simulink model "LoadTransferModel"  (R2026b)
settings: Solver=ode45  StopTime=1
undefined symbols (not defined in the file): Simulation, Vehicle
settings Model: DataDictionary=VehicleData.sldd  Creator=Xu Dingyi  LastModifiedBy=29358

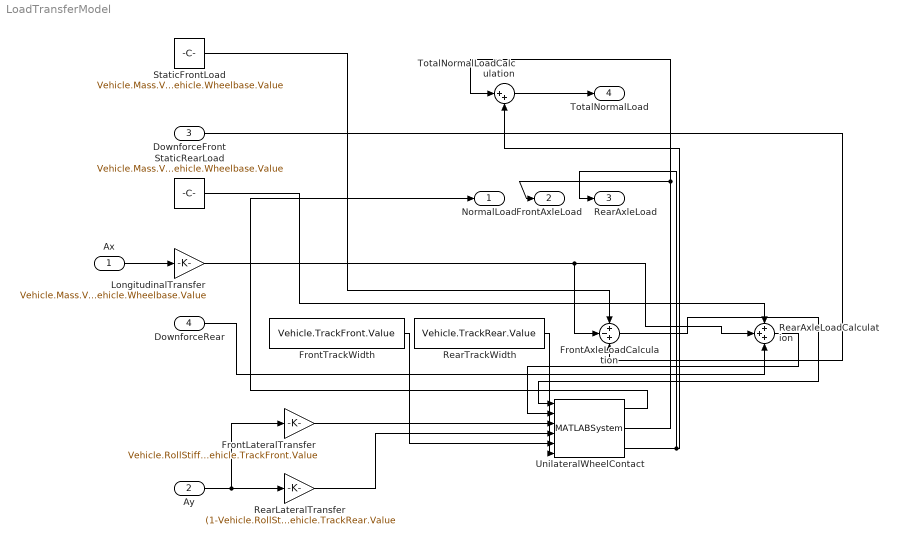
== system LoadTransferModel ==
  Ax : Inport  OutDataTypeStr=double  PortDimensions=1
  Ay : Inport  Port=2  OutDataTypeStr=double  PortDimensions=1
  DownforceFront : Inport  Port=3  OutDataTypeStr=double  PortDimensions=1
  DownforceRear : Inport  Port=4  OutDataTypeStr=double  PortDimensions=1
  FrontAxleLoadCalculation : Sum  Inputs=+-+
  FrontLateralTransfer : Gain  Gain=Vehicle.RollStiffnessDistributionFront.Value*Vehicle.Mass.Value*Vehicle.CGHeight.Value/Vehicle.TrackFront.Value
  FrontTrackWidth : Constant  Value=Vehicle.TrackFront.Value
  LongitudinalTransfer : Gain  Gain=Vehicle.Mass.Value*Vehicle.CGHeight.Value/Vehicle.Wheelbase.Value
  RearAxleLoadCalculation : Sum  Inputs=+++
  RearLateralTransfer : Gain  Gain=(1-Vehicle.RollStiffnessDistributionFront.Value)*Vehicle.Mass.Value*Vehicle.CGHeight.Value/Vehicle.TrackRear.Value
  RearTrackWidth : Constant  Value=Vehicle.TrackRear.Value
  StaticFrontLoad : Constant  Value=Vehicle.Mass.Value*Simulation.Gravity.Value*(Vehicle.Wheelbase.Value-Vehicle.CGToFrontAxle.Value)/Vehicle.Wheelbase.Value  OutDataTypeStr=double
  StaticRearLoad : Constant  Value=Vehicle.Mass.Value*Simulation.Gravity.Value*Vehicle.CGToFrontAxle.Value/Vehicle.Wheelbase.Value  OutDataTypeStr=double
  TotalNormalLoadCalculation : Sum  Inputs=|++
  UnilateralWheelContact : MATLABSystem  System=WheelNormalLoadDistributor  SimulateUsing=Code generation
      mask Type: WheelNormalLoadDistributor
  NormalLoad : Outport
  FrontAxleLoad : Outport  Port=2
  RearAxleLoad : Outport  Port=3
  TotalNormalLoad : Outport  Port=4
  wires:
  Ax/1 -> LongitudinalTransfer/1
  UnilateralWheelContact/3 -> TotalNormalLoadCalculation/2, RearAxleLoad/1
  UnilateralWheelContact/2 -> TotalNormalLoadCalculation/1, FrontAxleLoad/1
  UnilateralWheelContact/1 -> NormalLoad/1
  RearTrackWidth/1 -> UnilateralWheelContact/6
  FrontTrackWidth/1 -> UnilateralWheelContact/5
  RearLateralTransfer/1 -> UnilateralWheelContact/4
  FrontLateralTransfer/1 -> UnilateralWheelContact/3
  StaticFrontLoad/1 -> FrontAxleLoadCalculation/1
  LongitudinalTransfer/1 -> RearAxleLoadCalculation/2, FrontAxleLoadCalculation/2
  DownforceFront/1 -> FrontAxleLoadCalculation/3
  StaticRearLoad/1 -> RearAxleLoadCalculation/1
  DownforceRear/1 -> RearAxleLoadCalculation/3
  Ay/1 -> RearLateralTransfer/1, FrontLateralTransfer/1
  FrontAxleLoadCalculation/1 -> UnilateralWheelContact/1
  RearAxleLoadCalculation/1 -> UnilateralWheelContact/2
  TotalNormalLoadCalculation/1 -> TotalNormalLoad/1
